simulink model "drone_control_model"  (R2022b)
settings: Solver=VariableStepAuto  StartTime=0.0  StopTime=10.0  RelTol=1e-3
undefined symbols (not defined in the file): b, g, Ir, Ixx, Iyy, Izz, k, l, m, pitch_0, pitch_d, roll_0, roll_d, yaw_0, yaw_d, z_d
libraries: slpidlib x4
settings Model: Creator=mluser  LastModifiedBy=Gerardo

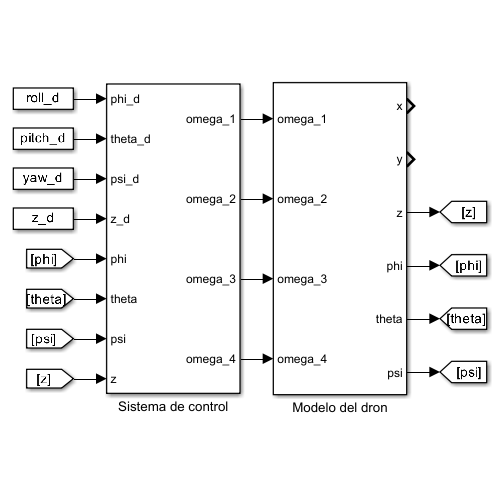
[thumbnail: Simulink's stored preview of the top-level diagram]
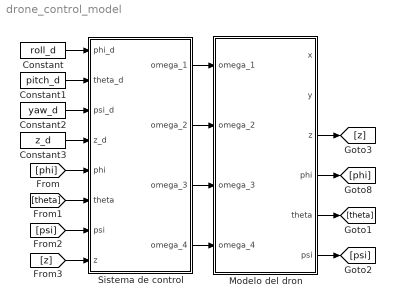
== system drone_control_model ==
  Constant : Constant  Value=roll_d
  Constant1 : Constant  Value=pitch_d
  Constant2 : Constant  Value=yaw_d
  Constant3 : Constant  Value=z_d
  Modelo del dron : Subsystem
  Sistema de control : Subsystem
  wires:
  Constant/1 -> Sistema de control/1(phi_d)
  Constant1/1 -> Sistema de control/2(theta_d)
  Constant2/1 -> Sistema de control/3(psi_d)
  Constant3/1 -> Sistema de control/4(z_d)
  Sistema de control/1(omega_1) -> Modelo del dron/1(omega_1)
  Sistema de control/2(omega_2) -> Modelo del dron/2(omega_2)
  Sistema de control/3(omega_3) -> Modelo del dron/3(omega_3)
  Sistema de control/4(omega_4) -> Modelo del dron/4(omega_4)
  Modelo del dron/4(phi) -> [phi]
  Modelo del dron/5(theta) -> [theta]
  Modelo del dron/6(psi) -> [psi]
  [phi] -> Sistema de control/5(phi)
  [theta] -> Sistema de control/6(theta)
  [psi] -> Sistema de control/7(psi)
  [z] -> Sistema de control/8(z)
  Modelo del dron/3(z) -> [z]

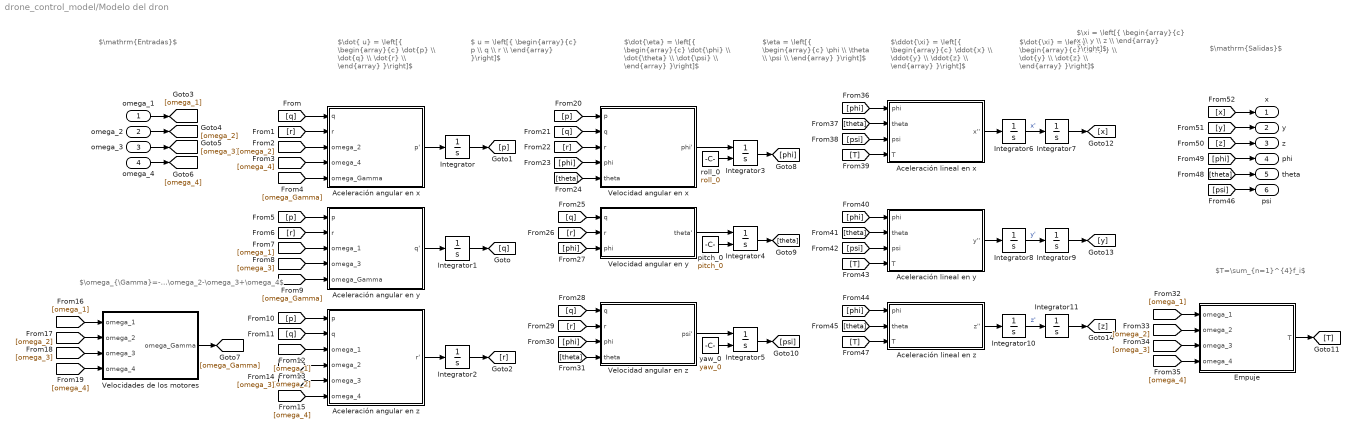
== system drone_control_model/Modelo del dron ==
  note: $\dot{\nu} = \left[{ \begin{array}{c} \dot{p} \\ \dot{q} \\ \dot{r} \\ \end{array} }\right]$
  note: $\nu = \left[{ \begin{array}{c} p \\ q \\ r \\ \end{array} }\right]$
  note: $\dot{\eta} = \left[{ \begin{array}{c} \dot{\phi} \\ \dot{\theta} \\ \dot{\psi} \\ \end{array} }\right]$
  note: $\eta = \left[{ \begin{array}{c} \phi \\ \theta \\ \psi \\ \end{array} }\right]$
  note: $\ddot{\xi} = \left[{ \begin{array}{c} \ddot{x} \\ \ddot{y} \\ \ddot{z} \\ \end{array} }\right]$
  note: $\dot{\xi} = \left[{ \begin{array}{c} \dot{x} \\ \dot{y} \\ \dot{z} \\ \end{array} }\right]$
  note: $\xi = \left[{ \begin{array}{c} x \\ y \\ z \\ \end{array} }\right]$
  note: $T=\sum_{n=1}^{4}f_i$
  note: $\omega_{\Gamma}=-\omega_1+\omega_2-\omega_3+\omega_4$
  note: $\mathrm{Entradas}$
  note: $\mathrm{Salidas}$
  omega_1 : Inport
  omega_2 : Inport  Port=2
  omega_3 : Inport  Port=3
  omega_4 : Inport  Port=4
  Aceleración angular en x : Subsystem
  Aceleración angular en y : Subsystem
  Aceleración angular en z : Subsystem
  Aceleración lineal en x : Subsystem
  Aceleración lineal en y : Subsystem
  Aceleración lineal en z : Subsystem
  Empuje : Subsystem
  Integrator{,1..2,6..11} (9 alike) : Integrator
  Integrator3 : Integrator  InitialConditionSource=external
  Integrator4 : Integrator  InitialConditionSource=external
  Integrator5 : Integrator  InitialConditionSource=external
  Velocidad angular en x : Subsystem
  Velocidad angular en y : Subsystem
  Velocidad angular en z : Subsystem
  Velocidades de los motores : Subsystem
  pitch_0 : Constant  Value=pitch_0
  roll_0 : Constant  Value=roll_0
  yaw_0 : Constant  Value=yaw_0
  x : Outport
  y : Outport  Port=2
  z : Outport  Port=3
  phi : Outport  Port=4
  theta : Outport  Port=5
  psi : Outport  Port=6
  wires:
  Aceleración angular en x/1(p') -> Integrator/1
  Aceleración angular en y/1(q') -> Integrator1/1
  Aceleración angular en z/1(r') -> Integrator2/1
  Velocidad angular en y/1(theta') -> Integrator4/1
  Velocidad angular en z/1(psi') -> Integrator5/1
  Velocidad angular en x/1(phi') -> Integrator3/1
  roll_0/1 -> Integrator3/2
  pitch_0/1 -> Integrator4/2
  yaw_0/1 -> Integrator5/2
  [q] -> Aceleración angular en x/1(q)
  Integrator1/1 -> [q]
  [r] -> Aceleración angular en x/2(r)
  [omega_2] -> Aceleración angular en x/3(omega_2)
  [omega_4] -> Aceleración angular en x/4(omega_4)
  [omega_Gamma] -> Aceleración angular en x/5(omega_Gamma)
  Integrator/1 -> [p]
  Integrator2/1 -> [r]
  [p] -> Aceleración angular en y/1(p)
  [r] -> Aceleración angular en y/2(r)
  [omega_1] -> Aceleración angular en y/3(omega_1)
  [omega_3] -> Aceleración angular en y/4(omega_3)
  [omega_Gamma] -> Aceleración angular en y/5(omega_Gamma)
  [p] -> Aceleración angular en z/1(p)
  [q] -> Aceleración angular en z/2(q)
  [omega_1] -> Aceleración angular en z/3(omega_1)
  [omega_2] -> Aceleración angular en z/4(omega_2)
  [omega_3] -> Aceleración angular en z/5(omega_3)
  [omega_4] -> Aceleración angular en z/6(omega_4)
  omega_1/1 -> [omega_1]
  omega_2/1 -> [omega_2]
  omega_3/1 -> [omega_3]
  omega_4/1 -> [omega_4]
  Velocidades de los motores/1(omega_Gamma) -> [omega_Gamma]
  [omega_3] -> Velocidades de los motores/3(omega_3)
  [omega_2] -> Velocidades de los motores/2(omega_2)
  [omega_1] -> Velocidades de los motores/1(omega_1)
  [omega_4] -> Velocidades de los motores/4(omega_4)
  [p] -> Velocidad angular en x/1(p)
  [r] -> Velocidad angular en x/3(r)
  [q] -> Velocidad angular en x/2(q)
  [theta] -> Velocidad angular en x/5(theta)
  [phi] -> Velocidad angular en x/4(phi)
  [phi] -> Velocidad angular en y/3(phi)
  [q] -> Velocidad angular en y/1(q)
  [r] -> Velocidad angular en y/2(r)
  [phi] -> Velocidad angular en z/3(phi)
  [q] -> Velocidad angular en z/1(q)
  [r] -> Velocidad angular en z/2(r)
  [theta] -> Velocidad angular en z/4(theta)
  Integrator3/1 -> [phi]
  Integrator4/1 -> [theta]
  Integrator5/1 -> [psi]
  [omega_3] -> Empuje/3(omega_3)
  [omega_2] -> Empuje/2(omega_2)
  [omega_4] -> Empuje/4(omega_4)
  [omega_1] -> Empuje/1(omega_1)
  Empuje/1(T) -> [T]
  Aceleración lineal en x/1(x'') -> Integrator6/1
  Integrator6/1 -> Integrator7/1  "x'"
  [theta] -> Aceleración lineal en x/2(theta)
  [phi] -> Aceleración lineal en x/1(phi)
  [psi] -> Aceleración lineal en x/3(psi)
  [T] -> Aceleración lineal en x/4(T)
  Integrator7/1 -> [x]
  Integrator8/1 -> Integrator9/1  "y'"
  [phi] -> Aceleración lineal en y/1(phi)
  Integrator9/1 -> [y]
  [theta] -> Aceleración lineal en y/2(theta)
  [psi] -> Aceleración lineal en y/3(psi)
  Aceleración lineal en y/1(y'') -> Integrator8/1
  [T] -> Aceleración lineal en y/4(T)
  [T] -> Aceleración lineal en z/3(T)
  Aceleración lineal en z/1(z'') -> Integrator10/1
  [theta] -> Aceleración lineal en z/2(theta)
  Integrator11/1 -> [z]
  [phi] -> Aceleración lineal en z/1(phi)
  Integrator10/1 -> Integrator11/1  "z'"
  [psi] -> psi/1
  [theta] -> theta/1
  [phi] -> phi/1
  [z] -> z/1
  [y] -> y/1
  [x] -> x/1

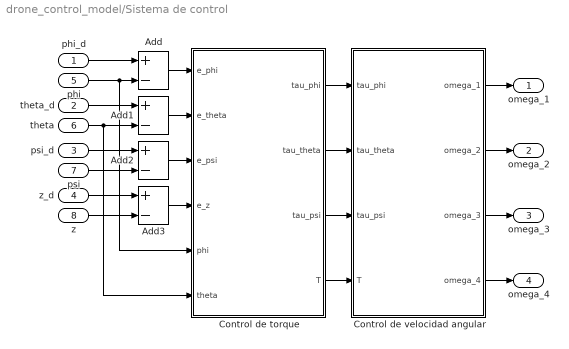
== system drone_control_model/Sistema de control ==
  phi_d : Inport
  theta_d : Inport  Port=2
  psi_d : Inport  Port=3
  z_d : Inport  Port=4
  phi : Inport  Port=5
  theta : Inport  Port=6
  psi : Inport  Port=7
  z : Inport  Port=8
  Add{,1..3} (4 alike) : Sum  Inputs=+-
  Control de torque : Subsystem
  Control de velocidad angular : Subsystem
  omega_1 : Outport
  omega_2 : Outport  Port=2
  omega_3 : Outport  Port=3
  omega_4 : Outport  Port=4
  wires:
  Control de torque/2(tau_theta) -> Control de velocidad angular/2(tau_theta)
  Control de torque/3(tau_psi) -> Control de velocidad angular/3(tau_psi)
  phi_d/1 -> Add/1
  phi/1 -> Control de torque/5(phi), Add/2
  theta_d/1 -> Add1/1
  theta/1 -> Control de torque/6(theta), Add1/2
  psi_d/1 -> Add2/1
  psi/1 -> Add2/2
  z/1 -> Add3/2
  z_d/1 -> Add3/1
  Add/1 -> Control de torque/1(e_phi)
  Add1/1 -> Control de torque/2(e_theta)
  Add2/1 -> Control de torque/3(e_psi)
  Add3/1 -> Control de torque/4(e_z)
  Control de velocidad angular/1(omega_1) -> omega_1/1
  Control de velocidad angular/2(omega_2) -> omega_2/1
  Control de velocidad angular/3(omega_3) -> omega_3/1
  Control de velocidad angular/4(omega_4) -> omega_4/1
  Control de torque/4(T) -> Control de velocidad angular/4(T)
  Control de torque/1(tau_phi) -> Control de velocidad angular/1(tau_phi)

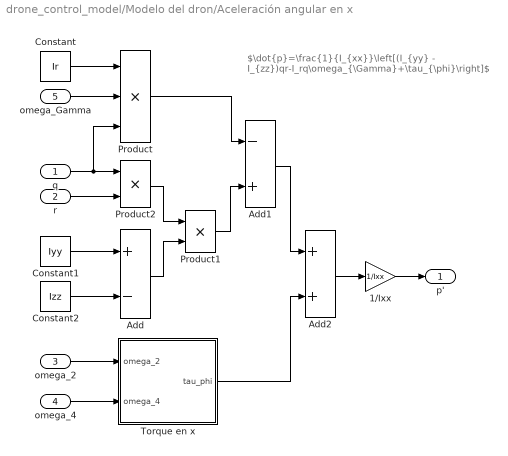
== system drone_control_model/Modelo del dron/Aceleración angular en x ==
  note: $\dot{p}=\frac{1}{I_{xx}}\left[(I_{yy} - I_{zz})qr-I_rq\omega_{\Gamma}+\tau_{\phi}\right]$
  q : Inport
  r : Inport  Port=2
  omega_2 : Inport  Port=3
  omega_4 : Inport  Port=4
  omega_Gamma : Inport  Port=5
  1/Ixx : Gain  Gain=1/Ixx
  Add : Sum  Inputs=+-
  Add1 : Sum  Inputs=-+
  Add2 : Sum
  Constant : Constant  Value=Ir
  Constant1 : Constant  Value=Iyy
  Constant2 : Constant  Value=Izz
  Product : Product  Inputs=3
  Product1 : Product
  Product2 : Product
  Torque en x : Subsystem
  p' : Outport
  wires:
  r/1 -> Product2/2
  q/1 -> Product/3, Product2/1
  omega_Gamma/1 -> Product/2
  Constant/1 -> Product/1
  Product2/1 -> Product1/1
  Constant1/1 -> Add/1
  Constant2/1 -> Add/2
  Add/1 -> Product1/2
  Product/1 -> Add1/1
  Product1/1 -> Add1/2
  omega_2/1 -> Torque en x/1(omega_2)
  omega_4/1 -> Torque en x/2(omega_4)
  Add1/1 -> Add2/1
  Torque en x/1(tau_phi) -> Add2/2
  Add2/1 -> 1/Ixx/1
  1/Ixx/1 -> p'/1

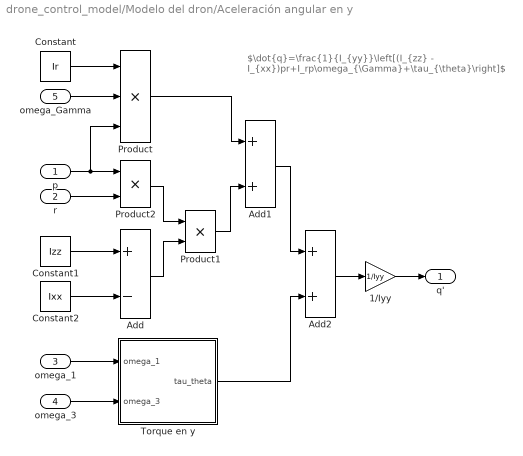
== system drone_control_model/Modelo del dron/Aceleración angular en y ==
  note: $\dot{q}=\frac{1}{I_{yy}}\left[(I_{zz} - I_{xx})pr+I_rp\omega_{\Gamma}+\tau_{\theta}\right]$
  p : Inport
  r : Inport  Port=2
  omega_1 : Inport  Port=3
  omega_3 : Inport  Port=4
  omega_Gamma : Inport  Port=5
  1/Iyy : Gain  Gain=1/Iyy
  Add : Sum  Inputs=+-
  Add1 : Sum
  Add2 : Sum
  Constant : Constant  Value=Ir
  Constant1 : Constant  Value=Izz
  Constant2 : Constant  Value=Ixx
  Product : Product  Inputs=3
  Product1 : Product
  Product2 : Product
  Torque en y : Subsystem
  q' : Outport
  wires:
  Constant/1 -> Product/1
  Product2/1 -> Product1/1
  Constant1/1 -> Add/1
  Constant2/1 -> Add/2
  Add/1 -> Product1/2
  Product/1 -> Add1/1
  Product1/1 -> Add1/2
  Add1/1 -> Add2/1
  Torque en y/1(tau_theta) -> Add2/2
  Add2/1 -> 1/Iyy/1
  1/Iyy/1 -> q'/1
  omega_Gamma/1 -> Product/2
  p/1 -> Product/3, Product2/1
  r/1 -> Product2/2
  omega_1/1 -> Torque en y/1(omega_1)
  omega_3/1 -> Torque en y/2(omega_3)

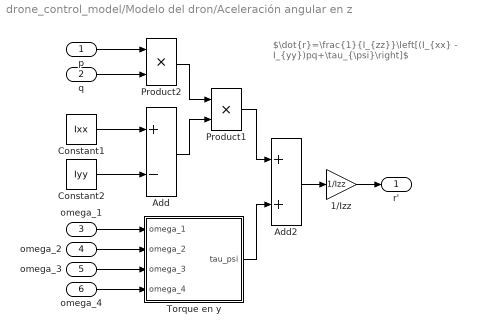
== system drone_control_model/Modelo del dron/Aceleración angular en z ==
  note: $\dot{r}=\frac{1}{I_{zz}}\left[(I_{xx} - I_{yy})pq+\tau_{\psi}\right]$
  p : Inport
  q : Inport  Port=2
  omega_1 : Inport  Port=3
  omega_2 : Inport  Port=4
  omega_3 : Inport  Port=5
  omega_4 : Inport  Port=6
  1/Izz : Gain  Gain=1/Izz
  Add : Sum  Inputs=+-
  Add2 : Sum
  Constant1 : Constant  Value=Ixx
  Constant2 : Constant  Value=Iyy
  Product1 : Product
  Product2 : Product
  Torque en y : Subsystem
  r' : Outport
  wires:
  Product2/1 -> Product1/1
  Constant1/1 -> Add/1
  Constant2/1 -> Add/2
  Add/1 -> Product1/2
  Torque en y/1(tau_psi) -> Add2/2
  Add2/1 -> 1/Izz/1
  1/Izz/1 -> r'/1
  p/1 -> Product2/1
  q/1 -> Product2/2
  omega_1/1 -> Torque en y/1(omega_1)
  omega_2/1 -> Torque en y/2(omega_2)
  Product1/1 -> Add2/1
  omega_3/1 -> Torque en y/3(omega_3)
  omega_4/1 -> Torque en y/4(omega_4)

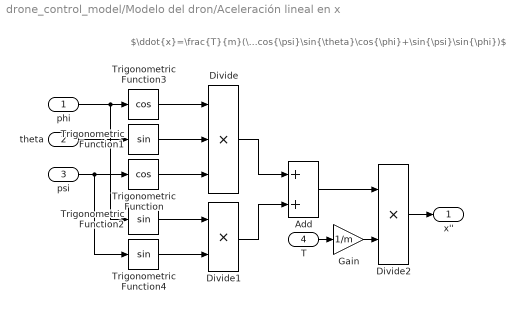
== system drone_control_model/Modelo del dron/Aceleración lineal en x ==
  note: $\ddot{x}=\frac{T}{m}(\cos{\psi}\sin{\theta}\cos{\phi}+\sin{\psi}\sin{\phi})$
  phi : Inport
  theta : Inport  Port=2
  psi : Inport  Port=3
  T : Inport  Port=4
  Add : Sum
  Divide : Product  Inputs=***
  Divide1 : Product  Inputs=**
  Divide2 : Product  Inputs=**
  Gain : Gain  Gain=1/m
  Trigonometric Function : Trigonometry  Operator=cos
  Trigonometric Function1 : Trigonometry
  Trigonometric Function2 : Trigonometry
  Trigonometric Function3 : Trigonometry  Operator=cos
  Trigonometric Function4 : Trigonometry
  x'' : Outport
  wires:
  Divide/1 -> Add/1
  phi/1 -> Trigonometric Function2/1, Trigonometric Function3/1
  theta/1 -> Trigonometric Function1/1
  psi/1 -> Trigonometric Function4/1, Trigonometric Function/1
  Trigonometric Function3/1 -> Divide/1
  Trigonometric Function1/1 -> Divide/2
  Trigonometric Function/1 -> Divide/3
  Trigonometric Function2/1 -> Divide1/1
  Trigonometric Function4/1 -> Divide1/2
  Divide1/1 -> Add/2
  Add/1 -> Divide2/1
  T/1 -> Gain/1
  Gain/1 -> Divide2/2
  Divide2/1 -> x''/1

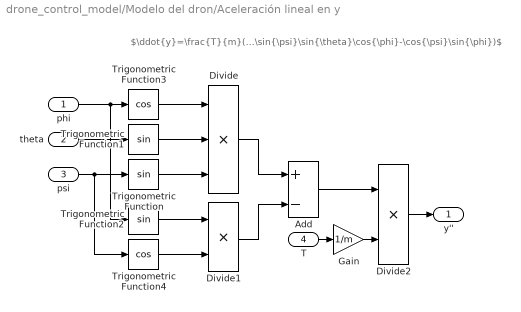
== system drone_control_model/Modelo del dron/Aceleración lineal en y ==
  note: $\ddot{y}=\frac{T}{m}(\sin{\psi}\sin{\theta}\cos{\phi}-\cos{\psi}\sin{\phi})$
  phi : Inport
  theta : Inport  Port=2
  psi : Inport  Port=3
  T : Inport  Port=4
  Add : Sum  Inputs=+-
  Divide : Product  Inputs=***
  Divide1 : Product  Inputs=**
  Divide2 : Product  Inputs=**
  Gain : Gain  Gain=1/m
  Trigonometric Function : Trigonometry
  Trigonometric Function1 : Trigonometry
  Trigonometric Function2 : Trigonometry
  Trigonometric Function3 : Trigonometry  Operator=cos
  Trigonometric Function4 : Trigonometry  Operator=cos
  y'' : Outport
  wires:
  Divide/1 -> Add/1
  phi/1 -> Trigonometric Function2/1, Trigonometric Function3/1
  theta/1 -> Trigonometric Function1/1
  psi/1 -> Trigonometric Function4/1, Trigonometric Function/1
  Trigonometric Function3/1 -> Divide/1
  Trigonometric Function1/1 -> Divide/2
  Trigonometric Function/1 -> Divide/3
  Trigonometric Function2/1 -> Divide1/1
  Trigonometric Function4/1 -> Divide1/2
  Divide1/1 -> Add/2
  Add/1 -> Divide2/1
  T/1 -> Gain/1
  Gain/1 -> Divide2/2
  Divide2/1 -> y''/1

== system drone_control_model/Modelo del dron/Aceleración lineal en z ==
  note: $\ddot{z}=-g+\frac{T}{m}(\cos{\theta}\cos{\phi})$
  phi : Inport
  theta : Inport  Port=2
  T : Inport  Port=3
  Add : Sum  Inputs=+-
  Constant : Constant  Value=g
  Divide : Product  Inputs=***
  Gain : Gain  Gain=1/m
  Trigonometric Function1 : Trigonometry  Operator=cos
  Trigonometric Function3 : Trigonometry  Operator=cos
  z'' : Outport
  wires:
  phi/1 -> Trigonometric Function3/1
  theta/1 -> Trigonometric Function1/1
  Trigonometric Function3/1 -> Divide/1
  Trigonometric Function1/1 -> Divide/2
  T/1 -> Gain/1
  Gain/1 -> Divide/3
  Divide/1 -> Add/1
  Constant/1 -> Add/2
  Add/1 -> z''/1

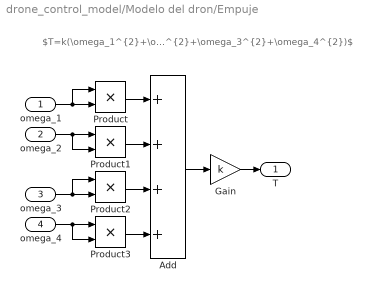
== system drone_control_model/Modelo del dron/Empuje ==
  note: $T=k(\omega_1^{2}+\omega_2^{2}+\omega_3^{2}+\omega_4^{2})$
  omega_1 : Inport
  omega_2 : Inport  Port=2
  omega_3 : Inport  Port=3
  omega_4 : Inport  Port=4
  Add : Sum  Inputs=++++
  Gain : Gain  Gain=k
  Product{,1..3} (4 alike) : Product
  T : Outport
  wires:
  Product3/1 -> Add/4
  omega_1/1 -> Product/1, Product/2
  Product/1 -> Add/1
  omega_2/1 -> Product1/2, Product1/1
  Gain/1 -> T/1
  omega_4/1 -> Product3/2, Product3/1
  Product2/1 -> Add/3
  omega_3/1 -> Product2/1, Product2/2
  Add/1 -> Gain/1
  Product1/1 -> Add/2

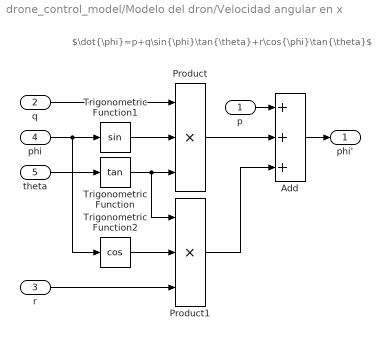
== system drone_control_model/Modelo del dron/Velocidad angular en x ==
  note: $\dot{\phi}=p+q\sin{\phi}\tan{\theta}+r\cos{\phi}\tan{\theta}$
  p : Inport
  q : Inport  Port=2
  r : Inport  Port=3
  phi : Inport  Port=4
  theta : Inport  Port=5
  Add : Sum  Inputs=+++
  Product : Product  Inputs=3
  Product1 : Product  Inputs=3
  Trigonometric Function : Trigonometry  Operator=tan
  Trigonometric Function1 : Trigonometry
  Trigonometric Function2 : Trigonometry  Operator=cos
  phi' : Outport
  wires:
  theta/1 -> Trigonometric Function/1
  phi/1 -> Trigonometric Function2/1, Trigonometric Function1/1
  Trigonometric Function1/1 -> Product/2
  Trigonometric Function/1 -> Product/3, Product1/1
  Trigonometric Function2/1 -> Product1/2
  r/1 -> Product1/3
  q/1 -> Product/1
  p/1 -> Add/1
  Product/1 -> Add/2
  Product1/1 -> Add/3
  Add/1 -> phi'/1

== system drone_control_model/Modelo del dron/Velocidad angular en y ==
  note: $\dot{\theta}=q\cos{\phi}-r\sin{\phi}$
  q : Inport
  r : Inport  Port=2
  phi : Inport  Port=3
  Add : Sum  Inputs=+-
  Product : Product
  Product1 : Product
  Trigonometric Function1 : Trigonometry  Operator=cos
  Trigonometric Function2 : Trigonometry
  theta' : Outport
  wires:
  phi/1 -> Trigonometric Function2/1, Trigonometric Function1/1
  q/1 -> Product/1
  Trigonometric Function1/1 -> Product/2
  r/1 -> Product1/2
  Trigonometric Function2/1 -> Product1/1
  Add/1 -> theta'/1
  Product/1 -> Add/1
  Product1/1 -> Add/2

== system drone_control_model/Modelo del dron/Velocidad angular en z ==
  note: $\dot{\psi}=q\frac{\sin{\phi}}{\cos{\theta}}+r\frac{\cos{\phi}}{\cos{\theta}}$
  q : Inport
  r : Inport  Port=2
  phi : Inport  Port=3
  theta : Inport  Port=4
  Add : Sum
  Divide : Product  Inputs=**/
  Divide1 : Product  Inputs=/**
  Trigonometric Function : Trigonometry  Operator=cos
  Trigonometric Function1 : Trigonometry
  Trigonometric Function2 : Trigonometry  Operator=cos
  psi' : Outport
  wires:
  theta/1 -> Trigonometric Function/1
  phi/1 -> Trigonometric Function2/1, Trigonometric Function1/1
  Trigonometric Function/1 -> Divide1/1, Divide/3
  Trigonometric Function1/1 -> Divide/2
  q/1 -> Divide/1
  Trigonometric Function2/1 -> Divide1/2
  r/1 -> Divide1/3
  Divide/1 -> Add/1
  Divide1/1 -> Add/2
  Add/1 -> psi'/1

== system drone_control_model/Modelo del dron/Velocidades de los motores ==
  omega_1 : Inport
  omega_2 : Inport  Port=2
  omega_3 : Inport  Port=3
  omega_4 : Inport  Port=4
  Sum : Sum  Inputs=+-+-
  omega_Gamma : Outport
  wires:
  omega_1/1 -> Sum/1
  omega_2/1 -> Sum/2
  omega_3/1 -> Sum/3
  omega_4/1 -> Sum/4
  Sum/1 -> omega_Gamma/1

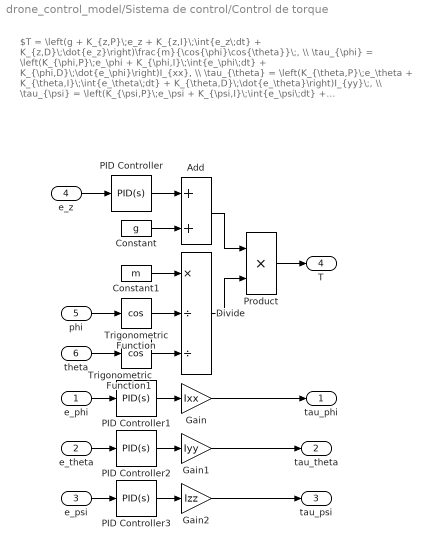
== system drone_control_model/Sistema de control/Control de torque ==
  note: $T = \left(g + K_{z,P}\;e_z + K_{z,I}\;\int{e_z\;dt} + K_{z,D}\;\dot{e_z}\right)\frac{m}{\cos{\phi}\cos{\theta}}\;, \\ \tau_{\phi} = \left(K_{\phi,P}\;e_\phi + K_{\phi,I}\;\int{e_\phi\;dt} + K_{\phi,D}\;\dot{e_\phi}\right)I_{xx}, \\ \tau_{\theta} = \left(K_{\theta,P}\;e_\theta + K_{\theta,I}\;\int{e_\theta\;dt} + K_{\theta,D}\;\dot{e_\theta}\right)I_{yy}\;, \\ \tau_{\psi} = \left(K_{\psi,P}\;e_\psi + K_{\psi,I}\;\int{e_\psi\;dt} + K_{\psi,D}\;\dot{e_\psi}\right)I_{zz}$
  e_phi : Inport
  e_theta : Inport  Port=2
  e_psi : Inport  Port=3
  e_z : Inport  Port=4
  phi : Inport  Port=5
  theta : Inport  Port=6
  Add : Sum
  Constant : Constant  Value=g
  Constant1 : Constant  Value=m
  Divide : Product  Inputs=*//
  Gain : Gain  Gain=Ixx
  Gain1 : Gain  Gain=Iyy
  Gain2 : Gain  Gain=Izz
  PID Controller : slpidlib/PID Controller  Controller=PID  Form=Parallel  TimeDomain=Continuous-time  UseExternalTs=off  SampleTime=-1  IntegratorMethod=Forward Euler  FilterMethod=Forward Euler  ControllerParametersSource=internal  P=57  I=0.001  UseKiTs=off  D=23  N=575  UseFilter=on  TunerSelectOption=Transfer Function Based (PID Tuner App)  InitialConditionSource=internal  InitialConditionForIntegrator=0  InitialConditionForFilter=0  DifferentiatorICPrevScaledInput=0  ExternalReset=none  TrackingMode=off  Kt=1  LimitOutput=on  SatLimitsSource=internal  UpperSaturationLimit=3  LowerSaturationLimit=-3  LinearizeAsGain=on  AntiWindupMode=none  Kb=1  LimitIntegrator=off  UpperIntegratorSaturationLimit=inf  LowerIntegratorSaturationLimit=-inf  POutMin=[]  POutMax=[]  IOutMin=[]  IOutMax=[]  DOutMin=[]  DOutMax=[]  NOutMin=[]  NOutMax=[]  SumOutMin=[]  SumOutMax=[]  SaturationOutMin=[]  SaturationOutMax=[]  PParamMin=[]  PParamMax=[]  IParamMin=[]  IParamMax=[]  DParamMin=[]  DParamMax=[]  NParamMin=[]  NParamMax=[]  KbParamMin=[]  KbParamMax=[]  KtParamMin=[]  KtParamMax=[]  KbOutMin=[]  KbOutMax=[]  KtOutMin=[]  KtOutMax=[]  IntegratorOutMin=[]  IntegratorOutMax=[]  FilterOutMin=[]  FilterOutMax=[]  SumI1OutMin=[]  SumI1OutMax=[]  SumI2OutMin=[]  SumI2OutMax=[]  SumI3OutMin=[]  SumI3OutMax=[]  SumI4OutMin=[]  SumI4OutMax=[]  SumDOutMin=[]  SumDOutMax=[]  DifferentiatorOutMin=[]  DifferentiatorOutMax=[]  FilterDiffOutCoefMin=[]  FilterDiffOutCoefMax=[]  ReciprocalOutMin=[]  ReciprocalOutMax=[]  SumDenOutMin=[]  SumDenOutMax=[]  SumNumOutMin=[]  SumNumOutMax=[]  DivideOutMin=[]  DivideOutMax=[]  UdiffTsProdOutMin=[]  UdiffTsProdOutMax=[]  NTsProdOutMin=[]  NTsProdOutMax=[]  UintegralTsProdOutMin=[]  UintegralTsProdOutMax=[]  UngainTsProdOutMin=[]  UngainTsProdOutMax=[]  ClampingZeroOutDataTypeStr=Inherit: Inherit via back propagation  ClampingZeroOutMin=[]  ClampingZeroOutMax=[]  FilterDenConstantOutDataTypeStr=Inherit: Inherit via back propagation  FilterDenConstantOutMin=[]  FilterDenConstantOutMax=[]  PCopyOutDataTypeStr=Inherit: Inherit via back propagation  PCopyOutMin=[]  PCopyOutMax=[]  NCopyOutDataTypeStr=Inherit: Inherit via back propagation  NCopyOutMin=[]  NCopyOutMax=[]  IntegratorContinuousStateAttributes=''  IntegratorStateMustResolveToSignalObject=off  IntegratorRTWStateStorageClass=Auto  FilterContinuousStateAttributes=''  FilterStateMustResolveToSignalObject=off  FilterRTWStateStorageClass=Auto  ParallelPVariant=InternalParameters  IdealPVariant=Disabled  IVariant=InternalParameters  DVariant=InternalParameters  IntegratorVariant=Continuous  SatVariant=Enabled  AWVariant=Passthrough  PCopyVariant=Disabled  TRVariant=Disabled  FdbkBlocksVariant=Forward  IdealPFdbkVariant=Disabled  SatFdbkVariant=Disabled  DerivativeFilterVariant=ContFilter  NVariant=InternalParameters  NCopyVariant=Disabled  FilterICVariant=InternalICsFilter  IntegratorICVariant=InternalICs  ExternalResetVariant=Disabled  TRSumVariant=Passthrough  SumFdbkVariant=Disabled  SumVariant=Sum_PID  TsampFilterVariant=InternalTs  TsampNgainVariant=Passthrough  TsampIntegralVariant=Passthrough  ExternalSaturationOutDataTypeStr=Inherit: Same as second input
  PID Controller1 : slpidlib/PID Controller  Controller=PID  Form=Parallel  TimeDomain=Continuous-time  UseExternalTs=off  SampleTime=-1  IntegratorMethod=Forward Euler  FilterMethod=Forward Euler  ControllerParametersSource=internal  P=55  I=0.01  UseKiTs=off  D=14.5  N=1415  UseFilter=on  TunerSelectOption=Transfer Function Based (PID Tuner App)  InitialConditionSource=internal  InitialConditionForIntegrator=0  InitialConditionForFilter=0  DifferentiatorICPrevScaledInput=0  ExternalReset=none  TrackingMode=off  Kt=1  LimitOutput=on  SatLimitsSource=internal  UpperSaturationLimit=3  LowerSaturationLimit=-3  LinearizeAsGain=on  AntiWindupMode=none  Kb=1  LimitIntegrator=off  UpperIntegratorSaturationLimit=inf  LowerIntegratorSaturationLimit=-inf  POutMin=[]  POutMax=[]  IOutMin=[]  IOutMax=[]  DOutMin=[]  DOutMax=[]  NOutMin=[]  NOutMax=[]  SumOutMin=[]  SumOutMax=[]  SaturationOutMin=[]  SaturationOutMax=[]  PParamMin=[]  PParamMax=[]  IParamMin=[]  IParamMax=[]  DParamMin=[]  DParamMax=[]  NParamMin=[]  NParamMax=[]  KbParamMin=[]  KbParamMax=[]  KtParamMin=[]  KtParamMax=[]  KbOutMin=[]  KbOutMax=[]  KtOutMin=[]  KtOutMax=[]  IntegratorOutMin=[]  IntegratorOutMax=[]  FilterOutMin=[]  FilterOutMax=[]  SumI1OutMin=[]  SumI1OutMax=[]  SumI2OutMin=[]  SumI2OutMax=[]  SumI3OutMin=[]  SumI3OutMax=[]  SumI4OutMin=[]  SumI4OutMax=[]  SumDOutMin=[]  SumDOutMax=[]  DifferentiatorOutMin=[]  DifferentiatorOutMax=[]  FilterDiffOutCoefMin=[]  FilterDiffOutCoefMax=[]  ReciprocalOutMin=[]  ReciprocalOutMax=[]  SumDenOutMin=[]  SumDenOutMax=[]  SumNumOutMin=[]  SumNumOutMax=[]  DivideOutMin=[]  DivideOutMax=[]  UdiffTsProdOutMin=[]  UdiffTsProdOutMax=[]  NTsProdOutMin=[]  NTsProdOutMax=[]  UintegralTsProdOutMin=[]  UintegralTsProdOutMax=[]  UngainTsProdOutMin=[]  UngainTsProdOutMax=[]  ClampingZeroOutDataTypeStr=Inherit: Inherit via back propagation  ClampingZeroOutMin=[]  ClampingZeroOutMax=[]  FilterDenConstantOutDataTypeStr=Inherit: Inherit via back propagation  FilterDenConstantOutMin=[]  FilterDenConstantOutMax=[]  PCopyOutDataTypeStr=Inherit: Inherit via back propagation  PCopyOutMin=[]  PCopyOutMax=[]  NCopyOutDataTypeStr=Inherit: Inherit via back propagation  NCopyOutMin=[]  NCopyOutMax=[]  IntegratorContinuousStateAttributes=''  IntegratorStateMustResolveToSignalObject=off  IntegratorRTWStateStorageClass=Auto  FilterContinuousStateAttributes=''  FilterStateMustResolveToSignalObject=off  FilterRTWStateStorageClass=Auto  ParallelPVariant=InternalParameters  IdealPVariant=Disabled  IVariant=InternalParameters  DVariant=InternalParameters  IntegratorVariant=Continuous  SatVariant=Enabled  AWVariant=Passthrough  PCopyVariant=Disabled  TRVariant=Disabled  FdbkBlocksVariant=Forward  IdealPFdbkVariant=Disabled  SatFdbkVariant=Disabled  DerivativeFilterVariant=ContFilter  NVariant=InternalParameters  NCopyVariant=Disabled  FilterICVariant=InternalICsFilter  IntegratorICVariant=InternalICs  ExternalResetVariant=Disabled  TRSumVariant=Passthrough  SumFdbkVariant=Disabled  SumVariant=Sum_PID  TsampFilterVariant=InternalTs  TsampNgainVariant=Passthrough  TsampIntegralVariant=Passthrough  ExternalSaturationOutDataTypeStr=Inherit: Same as second input
  PID Controller2 : slpidlib/PID Controller  Controller=PID  Form=Parallel  TimeDomain=Continuous-time  UseExternalTs=off  SampleTime=-1  IntegratorMethod=Forward Euler  FilterMethod=Forward Euler  ControllerParametersSource=internal  P=55  I=0.01  UseKiTs=off  D=11  N=1415  UseFilter=on  TunerSelectOption=Transfer Function Based (PID Tuner App)  InitialConditionSource=internal  InitialConditionForIntegrator=0  InitialConditionForFilter=0  DifferentiatorICPrevScaledInput=0  ExternalReset=none  TrackingMode=off  Kt=1  LimitOutput=on  SatLimitsSource=internal  UpperSaturationLimit=3  LowerSaturationLimit=-3  LinearizeAsGain=on  AntiWindupMode=none  Kb=1  LimitIntegrator=off  UpperIntegratorSaturationLimit=inf  LowerIntegratorSaturationLimit=-inf  POutMin=[]  POutMax=[]  IOutMin=[]  IOutMax=[]  DOutMin=[]  DOutMax=[]  NOutMin=[]  NOutMax=[]  SumOutMin=[]  SumOutMax=[]  SaturationOutMin=[]  SaturationOutMax=[]  PParamMin=[]  PParamMax=[]  IParamMin=[]  IParamMax=[]  DParamMin=[]  DParamMax=[]  NParamMin=[]  NParamMax=[]  KbParamMin=[]  KbParamMax=[]  KtParamMin=[]  KtParamMax=[]  KbOutMin=[]  KbOutMax=[]  KtOutMin=[]  KtOutMax=[]  IntegratorOutMin=[]  IntegratorOutMax=[]  FilterOutMin=[]  FilterOutMax=[]  SumI1OutMin=[]  SumI1OutMax=[]  SumI2OutMin=[]  SumI2OutMax=[]  SumI3OutMin=[]  SumI3OutMax=[]  SumI4OutMin=[]  SumI4OutMax=[]  SumDOutMin=[]  SumDOutMax=[]  DifferentiatorOutMin=[]  DifferentiatorOutMax=[]  FilterDiffOutCoefMin=[]  FilterDiffOutCoefMax=[]  ReciprocalOutMin=[]  ReciprocalOutMax=[]  SumDenOutMin=[]  SumDenOutMax=[]  SumNumOutMin=[]  SumNumOutMax=[]  DivideOutMin=[]  DivideOutMax=[]  UdiffTsProdOutMin=[]  UdiffTsProdOutMax=[]  NTsProdOutMin=[]  NTsProdOutMax=[]  UintegralTsProdOutMin=[]  UintegralTsProdOutMax=[]  UngainTsProdOutMin=[]  UngainTsProdOutMax=[]  ClampingZeroOutDataTypeStr=Inherit: Inherit via back propagation  ClampingZeroOutMin=[]  ClampingZeroOutMax=[]  FilterDenConstantOutDataTypeStr=Inherit: Inherit via back propagation  FilterDenConstantOutMin=[]  FilterDenConstantOutMax=[]  PCopyOutDataTypeStr=Inherit: Inherit via back propagation  PCopyOutMin=[]  PCopyOutMax=[]  NCopyOutDataTypeStr=Inherit: Inherit via back propagation  NCopyOutMin=[]  NCopyOutMax=[]  IntegratorContinuousStateAttributes=''  IntegratorStateMustResolveToSignalObject=off  IntegratorRTWStateStorageClass=Auto  FilterContinuousStateAttributes=''  FilterStateMustResolveToSignalObject=off  FilterRTWStateStorageClass=Auto  ParallelPVariant=InternalParameters  IdealPVariant=Disabled  IVariant=InternalParameters  DVariant=InternalParameters  IntegratorVariant=Continuous  SatVariant=Enabled  AWVariant=Passthrough  PCopyVariant=Disabled  TRVariant=Disabled  FdbkBlocksVariant=Forward  IdealPFdbkVariant=Disabled  SatFdbkVariant=Disabled  DerivativeFilterVariant=ContFilter  NVariant=InternalParameters  NCopyVariant=Disabled  FilterICVariant=InternalICsFilter  IntegratorICVariant=InternalICs  ExternalResetVariant=Disabled  TRSumVariant=Passthrough  SumFdbkVariant=Disabled  SumVariant=Sum_PID  TsampFilterVariant=InternalTs  TsampNgainVariant=Passthrough  TsampIntegralVariant=Passthrough  ExternalSaturationOutDataTypeStr=Inherit: Same as second input
  PID Controller3 : slpidlib/PID Controller  Controller=PID  Form=Parallel  TimeDomain=Continuous-time  UseExternalTs=off  SampleTime=-1  IntegratorMethod=Forward Euler  FilterMethod=Forward Euler  ControllerParametersSource=internal  P=53  I=0.04  UseKiTs=off  D=26  N=95  UseFilter=on  TunerSelectOption=Transfer Function Based (PID Tuner App)  InitialConditionSource=internal  InitialConditionForIntegrator=0  InitialConditionForFilter=0  DifferentiatorICPrevScaledInput=0  ExternalReset=none  TrackingMode=off  Kt=1  LimitOutput=on  SatLimitsSource=internal  UpperSaturationLimit=3  LowerSaturationLimit=-3  LinearizeAsGain=on  AntiWindupMode=none  Kb=1  LimitIntegrator=off  UpperIntegratorSaturationLimit=inf  LowerIntegratorSaturationLimit=-inf  POutMin=[]  POutMax=[]  IOutMin=[]  IOutMax=[]  DOutMin=[]  DOutMax=[]  NOutMin=[]  NOutMax=[]  SumOutMin=[]  SumOutMax=[]  SaturationOutMin=[]  SaturationOutMax=[]  PParamMin=[]  PParamMax=[]  IParamMin=[]  IParamMax=[]  DParamMin=[]  DParamMax=[]  NParamMin=[]  NParamMax=[]  KbParamMin=[]  KbParamMax=[]  KtParamMin=[]  KtParamMax=[]  KbOutMin=[]  KbOutMax=[]  KtOutMin=[]  KtOutMax=[]  IntegratorOutMin=[]  IntegratorOutMax=[]  FilterOutMin=[]  FilterOutMax=[]  SumI1OutMin=[]  SumI1OutMax=[]  SumI2OutMin=[]  SumI2OutMax=[]  SumI3OutMin=[]  SumI3OutMax=[]  SumI4OutMin=[]  SumI4OutMax=[]  SumDOutMin=[]  SumDOutMax=[]  DifferentiatorOutMin=[]  DifferentiatorOutMax=[]  FilterDiffOutCoefMin=[]  FilterDiffOutCoefMax=[]  ReciprocalOutMin=[]  ReciprocalOutMax=[]  SumDenOutMin=[]  SumDenOutMax=[]  SumNumOutMin=[]  SumNumOutMax=[]  DivideOutMin=[]  DivideOutMax=[]  UdiffTsProdOutMin=[]  UdiffTsProdOutMax=[]  NTsProdOutMin=[]  NTsProdOutMax=[]  UintegralTsProdOutMin=[]  UintegralTsProdOutMax=[]  UngainTsProdOutMin=[]  UngainTsProdOutMax=[]  ClampingZeroOutDataTypeStr=Inherit: Inherit via back propagation  ClampingZeroOutMin=[]  ClampingZeroOutMax=[]  FilterDenConstantOutDataTypeStr=Inherit: Inherit via back propagation  FilterDenConstantOutMin=[]  FilterDenConstantOutMax=[]  PCopyOutDataTypeStr=Inherit: Inherit via back propagation  PCopyOutMin=[]  PCopyOutMax=[]  NCopyOutDataTypeStr=Inherit: Inherit via back propagation  NCopyOutMin=[]  NCopyOutMax=[]  IntegratorContinuousStateAttributes=''  IntegratorStateMustResolveToSignalObject=off  IntegratorRTWStateStorageClass=Auto  FilterContinuousStateAttributes=''  FilterStateMustResolveToSignalObject=off  FilterRTWStateStorageClass=Auto  ParallelPVariant=InternalParameters  IdealPVariant=Disabled  IVariant=InternalParameters  DVariant=InternalParameters  IntegratorVariant=Continuous  SatVariant=Enabled  AWVariant=Passthrough  PCopyVariant=Disabled  TRVariant=Disabled  FdbkBlocksVariant=Forward  IdealPFdbkVariant=Disabled  SatFdbkVariant=Disabled  DerivativeFilterVariant=ContFilter  NVariant=InternalParameters  NCopyVariant=Disabled  FilterICVariant=InternalICsFilter  IntegratorICVariant=InternalICs  ExternalResetVariant=Disabled  TRSumVariant=Passthrough  SumFdbkVariant=Disabled  SumVariant=Sum_PID  TsampFilterVariant=InternalTs  TsampNgainVariant=Passthrough  TsampIntegralVariant=Passthrough  ExternalSaturationOutDataTypeStr=Inherit: Same as second input
  Product : Product
  Trigonometric Function : Trigonometry  Operator=cos
  Trigonometric Function1 : Trigonometry  Operator=cos
  tau_phi : Outport
  tau_theta : Outport  Port=2
  tau_psi : Outport  Port=3
  T : Outport  Port=4
  wires:
  PID Controller/1 -> Add/1
  Constant/1 -> Add/2
  phi/1 -> Trigonometric Function/1
  theta/1 -> Trigonometric Function1/1
  e_z/1 -> PID Controller/1
  Trigonometric Function1/1 -> Divide/3
  Trigonometric Function/1 -> Divide/2
  Constant1/1 -> Divide/1
  Add/1 -> Product/1
  Divide/1 -> Product/2
  Product/1 -> T/1
  e_phi/1 -> PID Controller1/1
  e_theta/1 -> PID Controller2/1
  e_psi/1 -> PID Controller3/1
  PID Controller1/1 -> Gain/1
  Gain/1 -> tau_phi/1
  PID Controller2/1 -> Gain1/1
  Gain1/1 -> tau_theta/1
  PID Controller3/1 -> Gain2/1
  Gain2/1 -> tau_psi/1

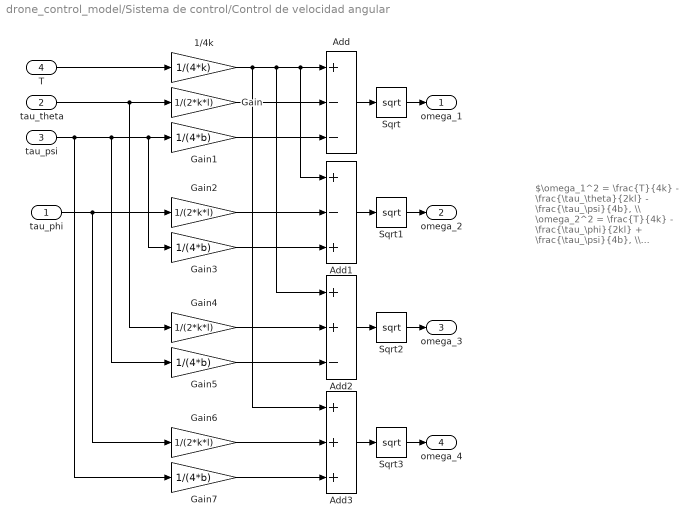
== system drone_control_model/Sistema de control/Control de velocidad angular ==
  note: $\omega_1^2 = \frac{T}{4k} - \frac{\tau_\theta}{2kl} - \frac{\tau_\psi}{4b}, \\ \omega_2^2 = \frac{T}{4k} - \frac{\tau_\phi}{2kl} + \frac{\tau_\psi}{4b}, \\ \omega_3^2 = \frac{T}{4k} + \frac{\tau_\theta}{2kl} - \frac{\tau_\psi}{4b}, \\ \omega_4^2 = \frac{T}{4k} + \frac{\tau_\phi}{2kl} + \frac{\tau_\psi}{4b}$
  tau_phi : Inport
  tau_theta : Inport  Port=2
  tau_psi : Inport  Port=3
  T : Inport  Port=4
  1/4k : Gain  Gain=1/(4*k)
  Add : Sum  Inputs=+--
  Add1 : Sum  Inputs=+-+
  Add2 : Sum  Inputs=++-
  Add3 : Sum  Inputs=+++
  Gain{,2,4,6} (4 alike) : Gain  Gain=1/(2*k*l)
  Gain{1,3,5,7} (4 alike) : Gain  Gain=1/(4*b)
  Sqrt{,1..3} (4 alike) : Sqrt
  omega_1 : Outport
  omega_2 : Outport  Port=2
  omega_3 : Outport  Port=3
  omega_4 : Outport  Port=4
  wires:
  T/1 -> 1/4k/1
  tau_theta/1 -> Gain/1, Gain4/1
  tau_psi/1 -> Gain7/1, Gain5/1, Gain3/1, Gain1/1
  1/4k/1 -> Add/1, Add1/1, Add2/1, Add3/1
  Gain/1 -> Add/2
  Gain1/1 -> Add/3
  Gain6/1 -> Add3/2
  Gain5/1 -> Add2/3
  Gain4/1 -> Add2/2
  Gain7/1 -> Add3/3
  Gain3/1 -> Add1/3
  Gain2/1 -> Add1/2
  tau_phi/1 -> Gain6/1, Gain2/1
  Add/1 -> Sqrt/1
  Sqrt/1 -> omega_1/1
  Add1/1 -> Sqrt1/1
  Add2/1 -> Sqrt2/1
  Add3/1 -> Sqrt3/1
  Sqrt1/1 -> omega_2/1
  Sqrt2/1 -> omega_3/1
  Sqrt3/1 -> omega_4/1

== system drone_control_model/Modelo del dron/Aceleración angular en x/Torque en x ==
  note: $\tau_{\phi}=lk(-\omega_2^{2}+\omega_4^{2})$
  omega_2 : Inport
  omega_4 : Inport  Port=2
  Add : Sum  Inputs=-+
  Gain : Gain  Gain=l*k
  Product : Product
  Product1 : Product
  tau_phi : Outport
  wires:
  omega_2/1 -> Product/1, Product/2
  omega_4/1 -> Product1/2, Product1/1
  Product/1 -> Add/1
  Product1/1 -> Add/2
  Add/1 -> Gain/1
  Gain/1 -> tau_phi/1

== system drone_control_model/Modelo del dron/Aceleración angular en y/Torque en y ==
  note: $\tau_{\theta}=lk(-\omega_1^{2}+\omega_3^{2})$
  omega_1 : Inport
  omega_3 : Inport  Port=2
  Add : Sum  Inputs=-+
  Gain : Gain  Gain=l*k
  Product : Product
  Product1 : Product
  tau_theta : Outport
  wires:
  omega_1/1 -> Product/1, Product/2
  omega_3/1 -> Product1/2, Product1/1
  Product/1 -> Add/1
  Product1/1 -> Add/2
  Add/1 -> Gain/1
  Gain/1 -> tau_theta/1

== system drone_control_model/Modelo del dron/Aceleración angular en z/Torque en y ==
  note: $\tau_{\psi}=b(-\omega_1^{2}+\omega_2^{2}-\omega_3^{2}+\omega_4^{2})$
  omega_1 : Inport
  omega_2 : Inport  Port=2
  omega_3 : Inport  Port=3
  omega_4 : Inport  Port=4
  Add : Sum  Inputs=-+-+
  Gain : Gain  Gain=b
  Product{,1..3} (4 alike) : Product
  tau_psi : Outport
  wires:
  omega_1/1 -> Product/1, Product/2
  omega_2/1 -> Product1/2, Product1/1
  Gain/1 -> tau_psi/1
  omega_3/1 -> Product2/1, Product2/2
  omega_4/1 -> Product3/2, Product3/1
  Product/1 -> Add/1
  Product1/1 -> Add/2
  Product2/1 -> Add/3
  Product3/1 -> Add/4
  Add/1 -> Gain/1
